simulink model "Transformation_matrices"  (R2021b)
settings: Solver=FixedStepDiscrete  StartTime=0.0  StopTime=1  FixedStep=Ts  RelTol=1e-3
InitFcn:
  | Ts=1e-5
undefined symbols (not defined in the file): DiscIntNeverNeededParam
libraries: spsPower3phInstantaneousLib x1
settings Model: Creator=lecci  LastModifiedBy=lecci

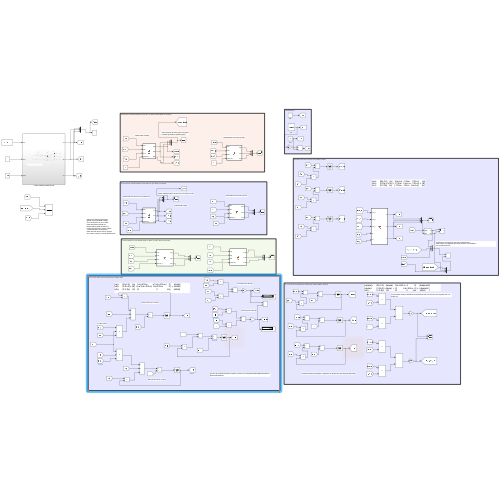
[thumbnail: Simulink's stored preview of the top-level diagram]
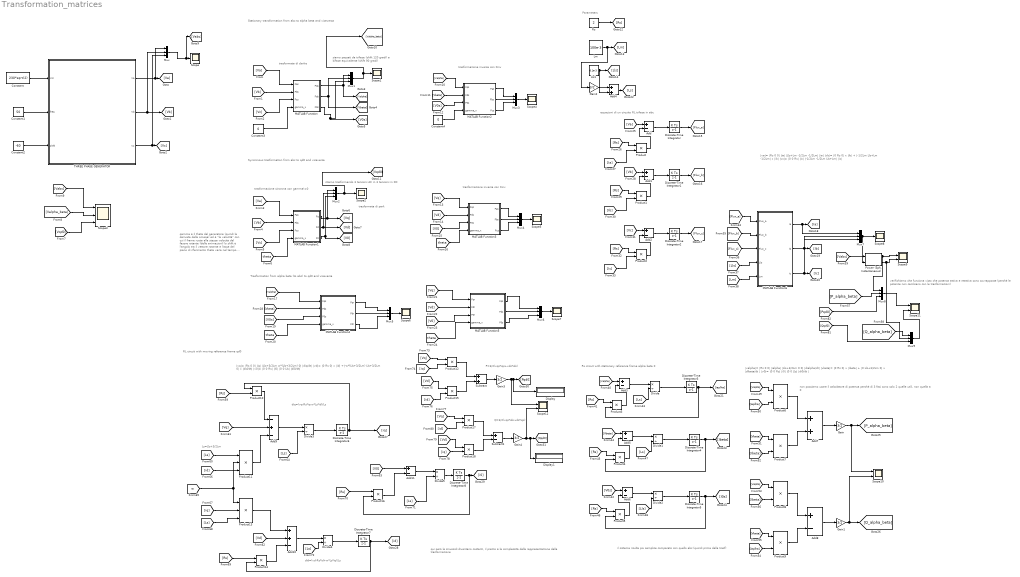
== system Transformation_matrices ==
  note: qui però le sinusoidi diventano costanti, il prezzo è la complessità della rappresentazione della trasformazione
  note: RL circuit with moving reference frame qd0
  note: Q=3/2(vqs*ids-vds*iqs)
  note: P=3/2(vqs*iqs+vds*ids)
  note: Ls=Lls+3/2Lm
  note: did=(vd-Rs*id+w*Ls*iq)/Ls
  note: diq=(vq-Rs*iq-w*Ls*id)/Ls
  note: |vq|= |Rs 0 0| |iq| |Lls+3/2Lm w*(Lls+3/2Lm) 0| |diq/dt|
      | |vd|= |0 Rs 0| x |id| +|-w*(Lls+3/2Lm) Lls+3/2Lm 0| x |did/dt|
      | |v0|= |0 0 Rs| |i0| |0 0 Lls| |di0/dt|
  note: il sistema risulta più semplice comparato con quello abc (quindi prima della trasf)
  note: |va|= |Rs 0 0| |ia| |Lls+Lm -1/2Lm -1/2Lm| |ia|
      | |vb|= |0 Rs 0| x |ib| + |-1/2Lm Lls+Lm -1/2Lm| x |ib|
      | |vc|= |0 0 Rs| |ic| |-1/2Lm -1/2Lm Lls+Lm| |ic|
  note: equazioni di un circuito RL trifase in abc
  note: verifichiamo che funziona visto che potenza attiva e
      | reattiva sono sovrapposte (perché le potenze non cambiano
      | con le trasformazioni)
  note: |valpha|= |Rs 0 0| |ialpha| |Lls+3/2Lm 0 0| |dialpha/dt|
      | |vbeta|= |0 Rs 0| x |ibeta| + |0 Lls+3/2Lm 0| x |dibeta/dt |
      | |v0|= |0 0 Rs| |i0| |0 0 Lls| |di0/dt |
  note: RL circuit with stationary reference frame alpha beta 0
  note: non possiamo usare il calcolatore di potenza perché di 3 fasi sono solo 2 quelle utili, non quella a 0
  note: Parameters
  note: Trasformation from alpha beta (to abc) to qd0 and viceversa
  note: Syncronous trasformation from abc to qd0 and viceversa
  note: Stationary transformation from abc to alpha beta and viceversa
  note: trasformazione inversa con Kinv
  note: trasformata di clarke
  note: trasformata di park
  note: stiamo trasformando 3 tensioni AC in 3 tensioni in DC
  note: gamma è il theta del generatore
      | (quindi la derivata della omega)
      | ed è "la velocità" con cui il frame
      | ruota alla stessa velocità del
      | fasore rotante (delle animazioni)
      | lo shift è l'angolo tra il vettore rotante
      | e l'asse del piano di riferimento
      | theta varia nel tempo. Esso è l'angolo
      | tra il vettore rotante e la linea dell'orizzonte
  note: trasformazione sincrona con gamma!=0
  note: siamo passati da trifase (shift 120 gradi)
      | a bifase equivalente (shift 90 gradi)
  note: trasformazione inversa con Kinv
  Add{,1..3,5..6,8,11} (8 alike) : Sum  Inputs=+-
  Add10 : Sum  Inputs=++-
  Add4 : Sum
  Add7 : Sum
  Add9 : Sum  Inputs=-+-
  Constant : Constant  Value=230*sqrt(2)
  Constant1 : Constant  Value=50
  Constant2 : Constant  Value=-60
  Constant3 : Constant  Value=0
  Constant4 : Constant  Value=0
  Discrete-Time Integrator{,1..8} (9 alike) : DiscreteIntegrator  SampleTime=-1  ICPrevOutput=DiscIntNeverNeededParam  ICPrevScaledInput=DiscIntNeverNeededParam
  Display : Display
  Display1 : Display
  Divide{,1..5} (6 alike) : Product  Inputs=*/
  Gain{,1..4} (5 alike) : Gain  Gain=3/2
  Lls1 : Constant  Value=0.1e-3
  Lm : Constant  Value=100e-3
  MATLAB Function : MATLAB Function  TreatAsAtomicUnit=on
  MATLAB Function1 : MATLAB Function  TreatAsAtomicUnit=on
  MATLAB Function2 : MATLAB Function  TreatAsAtomicUnit=on
  MATLAB Function3 : MATLAB Function  TreatAsAtomicUnit=on
  MATLAB Function4 : MATLAB Function  TreatAsAtomicUnit=on
  MATLAB Function5 : MATLAB Function  TreatAsAtomicUnit=on
  MATLAB Function6 : MATLAB Function  TreatAsAtomicUnit=on
  Mux{,1..9} (10 alike) : Mux  Inputs=3
  "Power (3ph, Instantaneous)" : spsPower3phInstantaneousLib/Power (3ph, Instantaneous)
  Product{,1..10,12,14..18} (17 alike) : Product
  Product11 : Product  Inputs=3
  Product13 : Product  Inputs=3
  Rs : Constant  Value=2
  Scope{,1..2,4..8} (8 alike) : Scope
  Scope{9..12} (4 alike) : Scope  NumInputPorts=2
  Scope3 : Scope  NumInputPorts=3
  Subtract : Sum
  Subtract1 : Sum  Inputs=+-
  THREE PHASE GENERATOR : Subsystem
  wires:
  Constant2/1 -> THREE PHASE GENERATOR/3(shift)
  Constant1/1 -> THREE PHASE GENERATOR/2(freq)
  Constant/1 -> THREE PHASE GENERATOR/1(Vm)
  THREE PHASE GENERATOR/1(Va) -> Mux/1, [Va]
  THREE PHASE GENERATOR/3(Vc) -> Mux/3, [Vc]
  THREE PHASE GENERATOR/2(Vb) -> Mux/2, [Vb]
  Mux/1 -> [Vabc], Scope/1
  [Va] -> MATLAB Function/1(Fas)
  [Vb] -> MATLAB Function/2(Fbs)
  [Vc] -> MATLAB Function/3(Fcs)
  Constant3/1 -> MATLAB Function/4(gamma_x)
  MATLAB Function/1(Fqs) -> [Valpha], Mux1/1
  MATLAB Function/2(Fds) -> [Vbeta], Mux1/2
  MATLAB Function/3(F0s) -> [V0s], Mux1/3
  Mux1/1 -> [Valpha_beta], Scope1/1
  [Vb] -> MATLAB Function1/2(Fbs)
  [Va] -> MATLAB Function1/1(Fas)
  MATLAB Function1/3(F0) -> [V0], Mux2/3
  [Vc] -> MATLAB Function1/3(Fcs)
  MATLAB Function1/2(Fd) -> [Vd], Mux2/2
  MATLAB Function1/1(Fq) -> [Vq], Mux2/1
  Mux2/1 -> [Vqd0], Scope2/1
  [theta] -> MATLAB Function1/4(gamma_x)
  [Valpha_beta] -> Scope3/2
  [Vabc] -> Scope3/1
  [Vqd0] -> Scope3/3
  [Valpha] -> MATLAB Function2/1(Fqs)
  [Vbeta] -> MATLAB Function2/2(Fds)
  [V0s] -> MATLAB Function2/3(F0s)
  Constant4/1 -> MATLAB Function2/4(gamma_x)
  Mux3/1 -> Scope4/1
  MATLAB Function2/1(Fas) -> Mux3/1
  MATLAB Function2/3(Fcs) -> Mux3/3
  MATLAB Function2/2(Fbs) -> Mux3/2
  MATLAB Function3/2(Fbs) -> Mux4/2
  Mux4/1 -> Scope5/1
  [Vq] -> MATLAB Function3/1(Fqs)
  [V0] -> MATLAB Function3/3(F0s)
  MATLAB Function3/1(Fas) -> Mux4/1
  MATLAB Function3/3(Fcs) -> Mux4/3
  [Vd] -> MATLAB Function3/2(Fds)
  [theta] -> MATLAB Function3/4(gamma_x)
  [Vbeta] -> MATLAB Function4/2(Fds)
  [theta] -> MATLAB Function4/4(gamma_x)
  [V0s] -> MATLAB Function4/3(F0s)
  [Valpha] -> MATLAB Function4/1(Fqs)
  MATLAB Function4/3(F0r) -> Mux5/3
  MATLAB Function4/1(Fqr) -> Mux5/1
  MATLAB Function4/2(Fdr) -> Mux5/2
  Mux5/1 -> Scope6/1
  [Vq] -> MATLAB Function5/1(Fqr)
  [Vd] -> MATLAB Function5/2(Fdr)
  [V0] -> MATLAB Function5/3(F0r)
  [theta] -> MATLAB Function5/4(gamma_x)
  Mux6/1 -> Scope7/1
  MATLAB Function5/3(F0s) -> Mux6/3
  MATLAB Function5/2(Fds) -> Mux6/2
  MATLAB Function5/1(Fqs) -> Mux6/1
  Rs/1 -> [Rs]
  Lm/1 -> Gain2/1, [Lm]
  [Va] -> Add/1
  [Rs] -> Product/1
  [Ia] -> Product/2
  Product/1 -> Add/2
  Add/1 -> Discrete-Time Integrator/1
  Discrete-Time Integrator/1 -> [Flux_a]
  Discrete-Time Integrator1/1 -> [Flux_b]
  Product1/1 -> Add1/2
  [Rs] -> Product1/1
  [Ib] -> Product1/2
  Add1/1 -> Discrete-Time Integrator1/1
  [Vb] -> Add1/1
  [Ic] -> Product2/2
  [Vc] -> Add2/1
  Add2/1 -> Discrete-Time Integrator2/1
  Product2/1 -> Add2/2
  Discrete-Time Integrator2/1 -> [Flux_c]
  [Rs] -> Product2/1
  [Flux_c] -> MATLAB Function6/3(Flux_c)
  [Flux_b] -> MATLAB Function6/2(Flux_b)
  [Flux_a] -> MATLAB Function6/1(Flux_a)
  [Lls] -> MATLAB Function6/4(Lls)
  [Lm] -> MATLAB Function6/5(Lm)
  MATLAB Function6/1(ia) -> Mux7/1, [Ia]
  MATLAB Function6/2(ib) -> Mux7/2, [Ib]
  MATLAB Function6/3(ic) -> Mux7/3, [Ic]
  Mux7/1 -> "Power (3ph, Instantaneous)"/2, Scope8/1
  [Vabc] -> "Power (3ph, Instantaneous)"/1
  "Power (3ph, Instantaneous)"/1 -> Mux8/1, Scope9/1
  "Power (3ph, Instantaneous)"/2 -> Scope9/2, Mux9/2
  Product3/1 -> Add3/2
  [Rs] -> Product3/1
  Discrete-Time Integrator3/1 -> Product3/2, [iaplha]
  [Valpha] -> Add3/1
  Add3/1 -> Divide/1
  [Ls] -> Divide/2
  Divide/1 -> Discrete-Time Integrator3/1
  [Ls] -> Divide1/2
  Discrete-Time Integrator4/1 -> Product4/2, [Ibeta]
  [Rs] -> Product4/1
  [Vbeta] -> Add5/1
  Divide1/1 -> Discrete-Time Integrator4/1
  Add5/1 -> Divide1/1
  Product4/1 -> Add5/2
  Divide2/1 -> Discrete-Time Integrator5/1
  [V0s] -> Add6/1
  Add6/1 -> Divide2/1
  [Rs] -> Product5/1
  Discrete-Time Integrator5/1 -> Product5/2, [I0s]
  [Lls] -> Divide2/2
  Product5/1 -> Add6/2
  [Valpha] -> Product6/1
  [iaplha] -> Product6/2
  [Vbeta] -> Product7/1
  [Ibeta] -> Product7/2
  Product6/1 -> Add7/1
  Product7/1 -> Add7/2
  Add7/1 -> Gain/1
  Gain/1 -> Scope10/1, [P_alpha_beta]
  [Vbeta] -> Product9/1
  Product8/1 -> Add8/1
  [Valpha] -> Product8/1
  Product9/1 -> Add8/2
  Add8/1 -> Gain1/1
  Gain1/1 -> Scope10/2, [Q_alpha_beta]
  [Ibeta] -> Product8/2
  [iaplha] -> Product9/2
  Add4/1 -> [Ls]
  Lls1/1 -> Add4/2, [Lls]
  Gain2/1 -> Add4/1
  Mux9/1 -> Scope11/2
  [Q_alpha_beta] -> Mux9/1
  Mux8/1 -> Scope11/1
  [P_alpha_beta] -> Mux8/2
  [Rs] -> Product10/2
  [Vq] -> Add9/2
  Product11/1 -> Add9/3
  Product10/1 -> Add9/1
  [Ls] -> Product11/1
  Add9/1 -> Divide3/1
  [Ls] -> Divide3/2
  [w] -> Product11/2, Product13/1
  [id] -> Product11/3
  Divide3/1 -> Discrete-Time Integrator6/1
  Discrete-Time Integrator6/1 -> Product10/1, [iq]
  [iq] -> Product13/2
  [Ls] -> Product13/3
  Product13/1 -> Add10/1
  [Vd] -> Add10/2
  Product14/1 -> Add10/3
  [Rs] -> Product14/1
  Add10/1 -> Divide4/1
  Divide4/1 -> Discrete-Time Integrator7/1
  Discrete-Time Integrator7/1 -> Product14/2, [id]
  [V0] -> Add11/1
  Product16/1 -> Add11/2
  [Rs] -> Product16/1
  Add11/1 -> Divide5/1
  [Ls] -> Divide5/2
  Divide5/1 -> Discrete-Time Integrator8/1
  Discrete-Time Integrator8/1 -> Product16/2, [i0]
  [Ls] -> Divide4/2
  [Vq] -> Product12/1
  [iq] -> Product12/2
  [Vd] -> Product15/1
  [id] -> Product15/2
  Product12/1 -> Subtract/1
  Product15/1 -> Subtract/2
  Subtract/1 -> Gain3/1
  Gain3/1 -> Scope12/1, Display/1, [Pqd0]
  Subtract1/1 -> Gain4/1
  Product17/1 -> Subtract1/1
  Gain4/1 -> Scope12/2, Display1/1, [Qqd0]
  Product18/1 -> Subtract1/2
  [Vd] -> Product18/1
  [Vq] -> Product17/1
  [id] -> Product17/2
  [iq] -> Product18/2
  [Qqd0] -> Mux9/3
  [Pqd0] -> Mux8/3

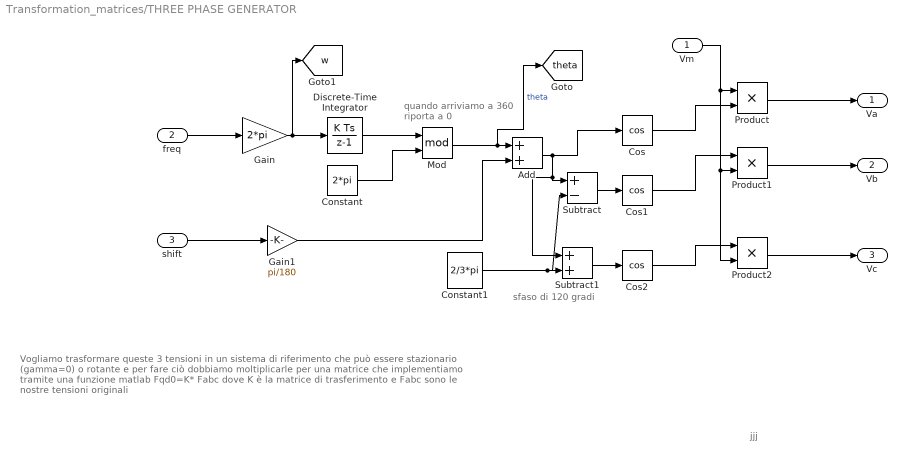
== system Transformation_matrices/THREE PHASE GENERATOR ==
  note: Vogliamo trasformare queste 3 tensioni in un sistema di riferimento che può essere stazionario (gamma=0) o rotante e per fare ciò dobbiamo moltiplicarle per una matrice che implementiamo tramite una funzione matlab
      | Fqd0=K* Fabc           dove K è la matrice di trasferimento e Fabc sono le nostre tensioni originali
  note: sfaso di 120 gradi
  note: jjj
  note: quando arriviamo a 360
      | riporta a 0
  Vm : Inport
  freq : Inport  Port=2
  shift : Inport  Port=3
  Add : Sum
  Constant : Constant  Value=2*pi
  Constant1 : Constant  Value=2/3*pi
  Cos : Trigonometry  Operator=cos
  Cos1 : Trigonometry  Operator=cos
  Cos2 : Trigonometry  Operator=cos
  Discrete-Time Integrator : DiscreteIntegrator  SampleTime=-1  ICPrevOutput=DiscIntNeverNeededParam  ICPrevScaledInput=DiscIntNeverNeededParam
  Gain : Gain  Gain=2*pi
  Gain1 : Gain  Gain=pi/180
  Mod : Math  Operator=mod  SaturateOnIntegerOverflow=on
  Product : Product
  Product1 : Product
  Product2 : Product
  Subtract : Sum  Inputs=+-
  Subtract1 : Sum
  Va : Outport
  Vb : Outport  Port=2
  Vc : Outport  Port=3
  tag scope: theta=global, w=global
  wires:
  freq/1 -> Gain/1
  Gain/1 -> [w], Discrete-Time Integrator/1
  Discrete-Time Integrator/1 -> Mod/1
  Constant/1 -> Mod/2
  Mod/1 -> [theta], Add/1  "theta"
  Add/1 -> Subtract1/1, Subtract/1, Cos/1
  Cos/1 -> Product/2
  Vm/1 -> Product2/2, Product1/2, Product/1
  Product/1 -> Va/1
  Cos1/1 -> Product1/1
  Cos2/1 -> Product2/1
  Product1/1 -> Vb/1
  Product2/1 -> Vc/1
  Subtract/1 -> Cos1/1
  Constant1/1 -> Subtract/2, Subtract1/2
  Subtract1/1 -> Cos2/1
  shift/1 -> Gain1/1
  Gain1/1 -> Add/2

== matlab function Transformation_matrices/MATLAB Function1 ==
  data: Fas input; Fq output; Fbs input; Fcs input; gamma_x input; Fd output; F0 output
function [Fq,Fd,F0] = fcn(Fas, Fbs, Fcs, gamma_x)
Fabcs=[Fas;Fbs;Fcs];
K=2/3*[cos(gamma_x) cos(gamma_x-2/3*pi) cos(gamma_x+pi*2/3);
       sin(gamma_x) sin(gamma_x-2/3*pi) sin(gamma_x+pi*2/3);
       1/2 1/2 1/2];

Fqd0=K*Fabcs;
Fq=Fqd0(1);
Fd=Fqd0(2);
F0=Fqd0(3);

end

== matlab function Transformation_matrices/MATLAB Function ==
  data: Fas input; Fqs output; Fbs input; Fcs input; gamma_x input; Fds output; F0s output
function [Fqs,Fds,F0s] = fcn(Fas, Fbs, Fcs, gamma_x)
Fabcs=[Fas;Fbs;Fcs]; %s sta per stazionarie
K=2/3*[cos(gamma_x) cos(gamma_x-2/3*pi) cos(gamma_x+pi*2/3);
       sin(gamma_x) sin(gamma_x-2/3*pi) sin(gamma_x+pi*2/3);
       1/2 1/2 1/2];

Fqd0s=K*Fabcs;
Fqs=Fqd0s(1);
Fds=Fqd0s(2);
F0s=Fqd0s(3);

end

== matlab function Transformation_matrices/MATLAB Function2 ==
  data: Fqs input; Fas output; Fds input; F0s input; gamma_x input; Fbs output; Fcs output
function [Fas, Fbs, Fcs] = fcn(Fqs,Fds,F0s,gamma_x)

Fqd0=[Fqs;Fds;F0s];

invK=[cos(gamma_x) sin(gamma_x) 1;
      cos(gamma_x-2*pi/3) sin(gamma_x-2/3*pi) 1;
      cos(gamma_x+2*pi/3) sin(gamma_x+2/3*pi) 1];
Fabc=invK*Fqd0;
Fas=Fabc(1);
Fbs=Fabc(2);
Fcs=Fabc(3);

== matlab function Transformation_matrices/MATLAB Function3 ==
  data: Fqs input; Fas output; Fds input; F0s input; gamma_x input; Fbs output; Fcs output
function [Fas, Fbs, Fcs] = fcn(Fqs,Fds,F0s,gamma_x)

Fqd0=[Fqs;Fds;F0s];

invK=[cos(gamma_x) sin(gamma_x) 1;
      cos(gamma_x-2*pi/3) sin(gamma_x-2/3*pi) 1;
      cos(gamma_x+2*pi/3) sin(gamma_x+2/3*pi) 1];
Fabc=invK*Fqd0;
Fas=Fabc(1);
Fbs=Fabc(2);
Fcs=Fabc(3);

== matlab function Transformation_matrices/MATLAB Function4 ==
  data: Fqs input; Fqr output; Fds input; F0s input; gamma_x input; Fdr output; F0r output
function [Fqr,Fdr,F0r]=fcn(Fqs,Fds,F0s,gamma_x)
Fqd0s=[Fqs;Fds;F0s];
R=[cos(gamma_x) -sin(gamma_x) 0;
    sin(gamma_x) cos(gamma_x) 0;
    0 0 1];
Fqd0r=R*Fqd0s;
Fqr=Fqd0r(1);
Fdr=Fqd0r(2);
F0r=Fqd0r(3);

== matlab function Transformation_matrices/MATLAB Function5 ==
  data: Fqr input; Fqs output; Fdr input; F0r input; gamma_x input; Fds output; F0s output
function [Fqs,Fds,F0s]=fcn(Fqr,Fdr,F0r,gamma_x)
Fqd0r=[Fqr;Fdr;F0r];
R=[cos(gamma_x) sin(gamma_x) 0;
    -sin(gamma_x) cos(gamma_x) 0;
    0 0 1];
Fqd0s=R*Fqd0r;
Fqs=Fqd0s(1);
Fds=Fqd0s(2);
F0s=Fqd0s(3);

== matlab function Transformation_matrices/MATLAB Function6 ==
  data: Flux_a input; ia output; Flux_b input; Flux_c input; ib output; ic output; Lls input; Lm input
function [ia,ib,ic]=fcn(Flux_a,Flux_b,Flux_c,Lls,Lm)
Flux_abc=[Flux_a;Flux_b;Flux_c];
L=[Lls+Lm -1/2*Lm -1/2*Lm;
   -1/2*Lm Lls+Lm -1/2*Lm;
   -1/2*Lm -1/2*Lm Lls+Lm];

Iabc=(L^-1)*Flux_abc;
ia=Iabc(1);
ib=Iabc(2);
ic=Iabc(3);
